simulink model "dynamics"  (R2021a)
settings: Solver=VariableStepAuto  StartTime=0.0  StopTime=10.0  RelTol=1e-3
settings Model: Creator=Wei Wu  LastModifiedBy=Wei Wu

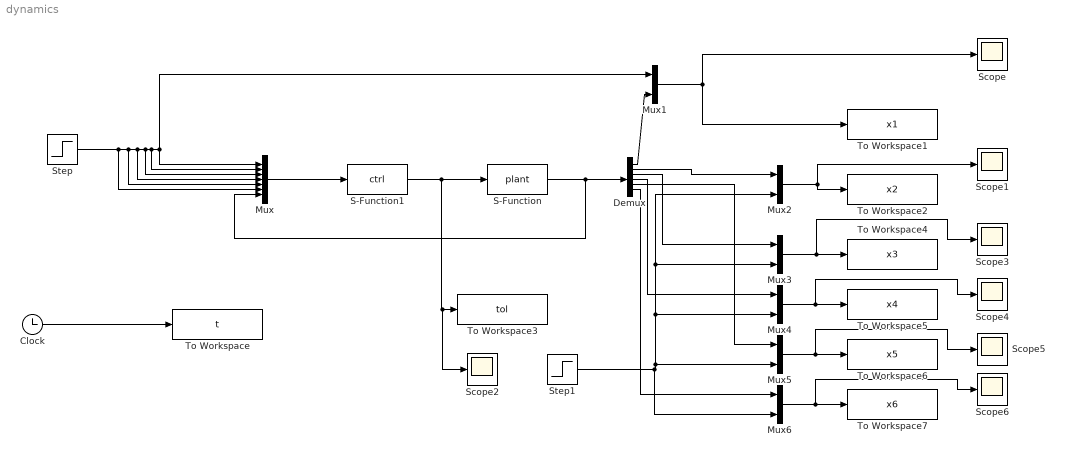
== system dynamics ==
  Clock : Clock
  Demux : Demux  Outputs=6
  Mux : Mux  Inputs=7
  Mux{1..6} (6 alike) : Mux  Inputs=2
  S-Function : S-Function  FunctionName=plant  SFunctionDeploymentMode=off  EnableBusSupport=off
  S-Function1 : S-Function  FunctionName=ctrl  SFunctionDeploymentMode=off  EnableBusSupport=off
  Scope{,1..6} (7 alike) : Scope
  Step : Step  SampleTime=0
  Step1 : Step  SampleTime=0
  To Workspace : ToWorkspace  VariableName=t  SaveFormat=Structure  SampleTime=-1
  To Workspace1 : ToWorkspace  VariableName=x1  SaveFormat=Structure  SampleTime=-1
  To Workspace2 : ToWorkspace  VariableName=x2  SaveFormat=Structure  SampleTime=-1
  To Workspace3 : ToWorkspace  VariableName=tol  SaveFormat=Structure  SampleTime=-1
  To Workspace4 : ToWorkspace  VariableName=x3  SaveFormat=Structure  SampleTime=-1
  To Workspace5 : ToWorkspace  VariableName=x4  SaveFormat=Structure  SampleTime=-1
  To Workspace6 : ToWorkspace  VariableName=x5  SaveFormat=Structure  SampleTime=-1
  To Workspace7 : ToWorkspace  VariableName=x6  SaveFormat=Structure  SampleTime=-1
  wires:
  Clock/1 -> To Workspace/1
  S-Function1/1 -> Scope2/1, To Workspace3/1, S-Function/1
  S-Function/1 -> Mux/7, Demux/1
  Mux/1 -> S-Function1/1
  Step/1 -> Mux/6, Mux/5, Mux/4, Mux/3, Mux/2, Mux1/1, Mux/1
  Demux/1 -> Mux1/2
  Demux/2 -> Mux2/1
  Mux1/1 -> Scope/1, To Workspace1/1
  Mux2/1 -> To Workspace2/1, Scope1/1
  Demux/3 -> Mux3/1
  Demux/4 -> Mux4/1
  Demux/5 -> Mux5/1
  Demux/6 -> Mux6/1
  Mux3/1 -> Scope3/1, To Workspace4/1
  Mux4/1 -> Scope4/1, To Workspace5/1
  Mux5/1 -> Scope5/1, To Workspace6/1
  Mux6/1 -> Scope6/1, To Workspace7/1
  Step1/1 -> Mux6/2, Mux4/2, Mux3/2, Mux2/2, Mux5/2
